simulink library "NeuroMuscularLibrary"  (R2019b)
settings: Solver=ode45  StartTime=0.0  StopTime=10.0  RelTol=1e-3  EnableMultiTasking=on
values from neighbouring files (symbols this model uses):
  a_18_19 = 116    [Prosthesis3R60Params.m]
  a_18_21 = 34    [Prosthesis3R60Params.m]
  a_2_3 = 18    [Prosthesis3R60Params.m]
  angle_offset = 0    [Prosthesis3R60Params.m]
  ankle_height = 0.08    [BodyMechParams.m]
  c = 0.05    [BodyMechParams.m]
  c_jointstop = 0.3 / (pi/180)    (= 17.1887338539)    [BodyMechParams.m]
  c_stance_comp_a0 = 885.0653    [Prosthesis3R60Params.m]
  c_stance_comp_a1 = 2.1443    [Prosthesis3R60Params.m]
  cg14 = 1/2*L14    (= 0.0475)    [Prosthesis3R60Params.m]
  cg25 = (5.45/11.05)*L25    (= 0.0379527149321)    [Prosthesis3R60Params.m]
  cg3 = (3.6/10.4)*L3    (= 0.0306346153846)    [Prosthesis3R60Params.m]
  d_fBall = 0.1    [BodyMechParams.m]
  d_fHeel = 0.05    [BodyMechParams.m]
  deltaLegAngleThr = 8*pi/180    (= 0.13962634016)    [CMGParams.m]
  DeltaThRef = 2e-3    (= 0.002)    [BodyMechParams.m]
  dt_visual = 0.001    [Prosthesis3R60Params.m]
  eref = 0.04    [BodyMechParams.m]
  Fmax = 4000    [MuscleEnergyTest.m]
  FmaxGLU = 1500    [BodyMechParams.m]
  footBallToAnkleDist = 0.16    [BodyMechParams.m]
  footBallToCenterDist = footLength/2    (= 0.1)    [BodyMechParams.m]
  footBallToHeelDist = footLength    (= 0.2)    [BodyMechParams.m]
  footCenterToCGDist = 0.14 - footBallToCenterDist    (= 0.04)    [BodyMechParams.m]
  footInertia = 0.005    [BodyMechParams.m]
  footLength = 0.2    [BodyMechParams.m]
  footMass = 1.25    [BodyMechParams.m]
  FT = 20    [MuscleEnergyTest.m]
  FT_GLU = 47.6    [BodyMechParams.m]
  g = 9.80665    [BodyMechParams.m]
  groundTheta = [atan(diff(groundZ)./diff(groundX)), 0]    [generateGround.m]
  groundZ = groundZ * stepSize/(largestStep+eps)    [generateGround.m]
  hatCenterToCGDist = 0.35 - hatHipToCenterDistLen    (= -0.05)    [BodyMechParams.m]
  hatHipToCenterDistLen = hatLength/2    (= 0.4)    [BodyMechParams.m]
  hatInertia = 3    [BodyMechParams.m]
  hatLeftHipToCenterDistWidth = .15    (= 0.15)    [BodyMechParams.m]
  hatLength = 0.8    [BodyMechParams.m]
  hatMass = 53.5    [BodyMechParams.m]
  hatThickness = 0.2    [BodyMechParams.m]
  hatWidth = 0.4    [BodyMechParams.m]
  J1011 = (4130)*1e-9    (= 4.13e-06)    [Prosthesis3R60Params.m]
  J1415 = (1.18*1e5)*1e-9    (= 0.000118)    [Prosthesis3R60Params.m]
  J18192021 = (6.86*1e4)*1e-9    (= 6.86e-05)    [Prosthesis3R60Params.m]
  J2526 = (3.59*1e4)*1e-9    (= 3.59e-05)    [Prosthesis3R60Params.m]
  J3467 = (25.96*1e4)*1e-9    (= 0.0002596)    [Prosthesis3R60Params.m]
  K = 5    [BodyMechParams.m]
  k_gn = k_gn/2    (= 39226.6)    [BodyMechParams.m]
  k_gt = k_gt/2    (= 39226.6)    [BodyMechParams.m]
  k_pressure = hatMass * g / DeltaThRef    (= 262327.8875)    [BodyMechParams.m]
  k_stance = 130000    [Prosthesis3R60Params.m]
  k_swing = 18750    [Prosthesis3R60Params.m]
  L0_stance = 0.08925    [Prosthesis3R60Params.m]
  L0_swing = 0.0896    [Prosthesis3R60Params.m]
  L10 = 7.9*1e-3    (= 0.0079)    [Prosthesis3R60Params.m]
  L11 = 3.3*1e-3    (= 0.0033)    [Prosthesis3R60Params.m]
  L14 = 95*1e-3    (= 0.095)    [Prosthesis3R60Params.m]
  L15 = 8.2*1e-3    (= 0.0082)    [Prosthesis3R60Params.m]
  L18 = 25.1*1e-3    (= 0.0251)    [Prosthesis3R60Params.m]
  L19 = 17.7*1e-3    (= 0.0177)    [Prosthesis3R60Params.m]
  L20 = 26*1e-3    (= 0.026)    [Prosthesis3R60Params.m]
  L21 = 1.7*1e-3    (= 0.0017)    [Prosthesis3R60Params.m]
  L25 = 76.95*1e-3    (= 0.07695)    [Prosthesis3R60Params.m]
  L26 = 2.8*1e-3    (= 0.0028)    [Prosthesis3R60Params.m]
  L3 = 88.5*1e-3    (= 0.0885)    [Prosthesis3R60Params.m]
  L4 = 1.7*1e-3    (= 0.0017)    [Prosthesis3R60Params.m]
  L6 = 40.25*1e-3    (= 0.04025)    [Prosthesis3R60Params.m]
  L7 = 14.9*1e-3    (= 0.0149)    [Prosthesis3R60Params.m]
  leg_l = [(thighLength - ankle_height/2) (shankLength - ankle_height/2)]    [BodyMechParams.m]
  legAngleSpeedMax = 10    [CMGParams.m]
  lopt = 0.055    [MuscleEnergyTest.m]
  loptBFSH = 0.12    [BodyMechParams.m]
  loptGAS = 0.05    [BodyMechParams.m]
  loptGLU = 0.11    [BodyMechParams.m]
  loptHAB = 0.09    [BodyMechParams.m]
  loptHAD = 0.10    (= 0.1)    [BodyMechParams.m]
  loptHAM = 0.10    (= 0.1)    [BodyMechParams.m]
  loptHFL = 0.11    [BodyMechParams.m]
  loptRF = 0.08    [BodyMechParams.m]
  loptSOL = 0.04    [BodyMechParams.m]
  loptTA = 0.06    [BodyMechParams.m]
  loptVAS = 0.08    [BodyMechParams.m]
  lslack = 0.245    [MuscleEnergyTest.m]
  lslackBFSH = 0.10    (= 0.1)    [BodyMechParams.m]
  lslackGAS = 0.40    (= 0.4)    [BodyMechParams.m]
  lslackGLU = 0.13    [BodyMechParams.m]
  lslackHAB = 0.07    [BodyMechParams.m]
  lslackHAD = 0.18    [BodyMechParams.m]
  lslackHAM = 0.31    [BodyMechParams.m]
  lslackHFL = 0.10    (= 0.1)    [BodyMechParams.m]
  lslackRF = 0.35    [BodyMechParams.m]
  lslackSOL = 0.26    [BodyMechParams.m]
  lslackTA = 0.24    [BodyMechParams.m]
  lslackVAS = 0.23    [BodyMechParams.m]
  m1011 = 49.5*1e-3    (= 0.0495)    [Prosthesis3R60Params.m]
  m1415 = 123.8*1e-3    (= 0.1238)    [Prosthesis3R60Params.m]
  m18192021 = 196.6*1e-3    (= 0.1966)    [Prosthesis3R60Params.m]
  m2526 = 58.3*1e-3    (= 0.0583)    [Prosthesis3R60Params.m]
  m3467 = 253.3*1e-3    (= 0.2533)    [Prosthesis3R60Params.m]
  mu_slide = 0.8    [BodyMechParams.m]
  mu_stick = 0.9    [BodyMechParams.m]
  N = 1.5    [BodyMechParams.m]    (also in cmaes.m = size(x,1); mergeCompareEnergyCosts.m = {S.name})
  phiKneeUpLimit = 5*pi/180    (= 0.0872664625997)    [BodyMechParams.m]
  phimaxGASa = (100-90)*pi/180    (= 0.174532925199)    [BodyMechParams.m]
  phimaxGASk = (180-140)*pi/180    (= 0.698131700798)    [BodyMechParams.m]
  phimaxRFk = (180-165)*pi/180    (= 0.261799387799)    [BodyMechParams.m]
  phimaxSOL = (100-90)*pi/180    (= 0.174532925199)    [BodyMechParams.m]
  phimaxTA = (80-90)*pi/180    (= -0.174532925199)    [BodyMechParams.m]
  phimaxVAS = (180-165)*pi/180    (= 0.261799387799)    [BodyMechParams.m]
  phirefBFSH = (180-160)*pi/180    (= 0.349065850399)    [BodyMechParams.m]
  phirefGASa = (80-90)*pi/180    (= -0.174532925199)    [BodyMechParams.m]
  phirefGASk = (180-165)*pi/180    (= 0.261799387799)    [BodyMechParams.m]
  phirefGLU = (120-180)*pi/180    (= -1.0471975512)    [BodyMechParams.m]
  phirefHAB = 10*pi/180    (= 0.174532925199)    [BodyMechParams.m]
  phirefHAD = 15*pi/180    (= 0.261799387799)    [BodyMechParams.m]
  phirefHAMh = (150-180)*pi/180    (= -0.523598775598)    [BodyMechParams.m]
  phirefHAMk = (180-180)*pi/180    (= 0)    [BodyMechParams.m]
  phirefHFL = (160-180)*pi/180    (= -0.349065850399)    [BodyMechParams.m]
  phirefRFh = (170-180)*pi/180    (= -0.174532925199)    [BodyMechParams.m]
  phirefRFk = (180-125)*pi/180    (= 0.959931088597)    [BodyMechParams.m]
  phirefSOL = (90-90)*pi/180    (= 0)    [BodyMechParams.m]
  ... (+64 more)
undefined symbols (not defined in the file or in its folder): ankleBackDriveGain, ankleCJointstop, ankleDgain, ankleFilterPID, ankleFilterSEA, ankleGearEff, ankleGearRatio, ankleIgain, ankleInitialAngle, ankleInputMass, ankleIntCoulomb, ankleIntDamping, ankleIntStatic, ankleParallelSpringDamping, ankleParallelSpringOffset, ankleParallelSpringStiffness, anklePgain, anklePlantarLimit, ankleSEADamping, ankleSEAStiffness, ankleTendonMass, ankleWMaxJointstop, D12_F, D12_S, D12_T, D12z_T, D13_F, D1G_F, D1G_HAT, D1G_S, D1G_T, D1Gy_F, DeltaS, DeltaSGLU, DeltaSHFL, dryFrictionDamping, dryFrictionStiffness, dryFrictionVelThresh, footMassp, FourBarL1, FourBarL3, GainDphiHATGLUst, GainDphiHATHABst, GainDphiHATHADst, GainDphiHATHFLst, GainFGASst, GainFGLUst, GainFHABst, GainFHAMst, GainFSOLst, GainFSOLTAst, GainFVASst, GainGAS, GainGLU, GainGLUswing, GainHAM, GainHAMHFL ... (+194)
libraries: sm_lib x332, nesl_utility x156, simulink x33, dspswit3 x30, $bdroot x19, simulink_extras x7
(part 7 of 15)

== system NeuroMuscularLibrary/Shanks ==
  CS2_to_knee : sm_lib/Frames and Transforms/Rigid Transform  TranslationMethod=Cartesian  TranslationStandardOffset=0  TranslationLengthUnit=m  TranslationStandardAxis=+Z  TranslationCartesianOffset=[D12_S 0 0]  TranslationROffset=0  TranslationROffsetUnits=m  TranslationZOffset=0  TranslationZOffsetUnits=m  TranslationThetaOffset=0  TranslationThetaOffsetUnits=deg  RotationMethod=None  RotationAngleUnits=deg  RotationStandardAxis=+Z  RotationAngle=0.0  RotationArbitraryAxis=[0 0 1]  FollAlignAxisA=+X  BaseAlignAxisA=+Y  FollAlignAxisB=+Y  BaseAlignAxisB=+Z  RotationSequenceAxes=FollowerAxes  RotationSequence=XYX  RotationSequenceAngles=[0 0 0]  RotationSequenceAnglesUnits=deg  RotationMatrix=[1 0 0; 0 1 0; 0 0 1]
  Cylindrical Solid : sm_lib/Body Elements/Cylindrical Solid  GraphicAmbientColor=[0.15 0.15 0.15 1.0]  BasedOnType=Mass  CenterOfMass=[0 0 0]  CenterOfMassUnits=m  GraphicDiffuseColor=[0.5 0.5 0.5]  CylinderLength=D12_S  CylinderLengthUnits=m  CylinderRadius=.04  CylinderRadiusUnits=m  Density=0  DensityUnits=kg/m^3  DoExposeReferenceFrame=on  GraphicEmissiveColor=[0.0 0.0 0.0 1.0]  ExportEntireGeometry=off  SerializedFrames=<Frames/>  MarkerShape=Sphere  MarkerSize=10  GraphicType=FromGeometry  InertiaType=CalculateFromGeometry  Mass=0  MassUnits=kg  MomentsOfInertia=[1 1 1]  MomentsOfInertiaUnits=kg*m^2  GraphicOpacity=1.0  ProductsOfInertia=[0 0 0]  ProductsOfInertiaUnits=kg*m^2  GraphicShininess=75  GraphicSpecularColor=[0.5 0.5 0.5 1.0]  GraphicVisPropType=SimpleVisualProperties
  Inertia : sm_lib/Body Elements/Inertia  InertiaType=Custom  Mass=m_S  MassUnits=kg  CenterOfMass=[0 0 0]  CenterOfMassUnits=m  MomentsOfInertia=[Inx_S Iny_S In_S]  MomentsOfInertiaUnits=kg*m^2  ProductsOfInertia=[0 0 0]  ProductsOfInertiaUnits=kg*m^2  GraphicType=None  MarkerShape=Inertia  MarkerSize=20  GraphicVisPropType=SimpleVisualProperties  GraphicDiffuseColor=[0.5 0.5 0.5]  GraphicSpecularColor=[0.5 0.5 0.5 1.0]  GraphicAmbientColor=[0.15 0.15 0.15 1.0]  GraphicEmissiveColor=[0.0 0.0 0.0 1.0]  GraphicShininess=75  GraphicOpacity=1.0
  Mux : Mux  Inputs=3
  Mux1 : Mux  Inputs=3
  PS-Simulink Converter{,1..5} (6 alike) : nesl_utility/PS-Simulink Converter  PhysicalDomain=network_engine_domain  SubClassName=ps_output  LeftPortType=input  RightPortType=output  PseudoPeriodic=off  Frequencies=[]  Unit=m  AffineConversion=off
  Reference Frame : sm_lib/Frames and Transforms/Reference Frame
  TO: X-forward Y-up Z-lateral : sm_lib/Frames and Transforms/Rigid Transform  TranslationMethod=StandardAxis  TranslationStandardOffset=D12z_T/2  TranslationLengthUnit=m  TranslationStandardAxis=+Y  TranslationCartesianOffset=[0 0 0]  TranslationROffset=0  TranslationROffsetUnits=m  TranslationZOffset=0  TranslationZOffsetUnits=m  TranslationThetaOffset=0  TranslationThetaOffsetUnits=deg  RotationMethod=AlignedAxes  RotationAngleUnits=deg  RotationStandardAxis=+Z  RotationAngle=0  RotationArbitraryAxis=[0 0 1]  FollAlignAxisA=+Z  BaseAlignAxisA=-Y  FollAlignAxisB=+X  BaseAlignAxisB=+X  RotationSequenceAxes=FollowerAxes  RotationSequence=XYX  RotationSequenceAngles=[0 0 0]  RotationSequenceAnglesUnits=deg  RotationMatrix=[1 0 0; 0 1 0; 0 0 1]
  To CG : sm_lib/Frames and Transforms/Rigid Transform  TranslationMethod=Cartesian  TranslationStandardOffset=0  TranslationLengthUnit=m  TranslationStandardAxis=+Z  TranslationCartesianOffset=[D1G_S 0 0]  TranslationROffset=0  TranslationROffsetUnits=m  TranslationZOffset=0  TranslationZOffsetUnits=m  TranslationThetaOffset=0  TranslationThetaOffsetUnits=deg  RotationMethod=None  RotationAngleUnits=deg  RotationStandardAxis=+Z  RotationAngle=0.0  RotationArbitraryAxis=[0 0 1]  FollAlignAxisA=+X  BaseAlignAxisA=+Y  FollAlignAxisB=+Y  BaseAlignAxisB=+Z  RotationSequenceAxes=FollowerAxes  RotationSequence=XYX  RotationSequenceAngles=[0 0 0]  RotationSequenceAnglesUnits=deg  RotationMatrix=[1 0 0; 0 1 0; 0 0 1]
  To center : sm_lib/Frames and Transforms/Rigid Transform  TranslationMethod=Cartesian  TranslationStandardOffset=0  TranslationLengthUnit=m  TranslationStandardAxis=+Z  TranslationCartesianOffset=[D12_S/2 0 0]  TranslationROffset=0  TranslationROffsetUnits=m  TranslationZOffset=0  TranslationZOffsetUnits=m  TranslationThetaOffset=0  TranslationThetaOffsetUnits=deg  RotationMethod=AlignedAxes  RotationAngleUnits=deg  RotationStandardAxis=+Z  RotationAngle=0.0  RotationArbitraryAxis=[0 0 1]  FollAlignAxisA=+Z  BaseAlignAxisA=+X  FollAlignAxisB=+Y  BaseAlignAxisB=+Y  RotationSequenceAxes=FollowerAxes  RotationSequence=XYX  RotationSequenceAngles=[0 0 0]  RotationSequenceAnglesUnits=deg  RotationMatrix=[1 0 0; 0 1 0; 0 0 1]
  Transform Sensor : sm_lib/Frames and Transforms/Transform Sensor  MeasurementFrame=NonRotatingBase  SenseAngle=off  SenseAxis=off  SenseAngle1=off  SenseAngle2=off  SenseAngle3=off  SenseQ=off  SenseR=off  SenseOmegaX=off  SenseOmegaY=off  SenseOmegaZ=off  SenseOmega1=off  SenseOmega2=off  SenseOmega3=off  SenseQDot=off  SenseRDot=off  SenseAlphaX=off  SenseAlphaY=off  SenseAlphaZ=off  SenseAlpha1=off  SenseAlpha2=off  SenseAlpha3=off  SenseQDDot=off  SenseRDDot=off  SenseX=on  SenseY=on  SenseZ=on  SenseRad=off  SenseAzim=off  SenseDist=off  SenseInc=off  SenseXDot=off  SenseYDot=off  SenseZDot=off  SenseRadDot=off  SenseAzimDot=off  SenseDistDot=off  SenseIncDot=off  SenseXDDot=off  SenseYDDot=off  SenseZDDot=off  SenseRadDDot=off  SenseAzimDDot=off  SenseDistDDot=off  SenseIncDDot=off
  Transform Sensor1 : sm_lib/Frames and Transforms/Transform Sensor  MeasurementFrame=NonRotatingBase  SenseAngle=off  SenseAxis=off  SenseAngle1=off  SenseAngle2=off  SenseAngle3=off  SenseQ=off  SenseR=off  SenseOmegaX=off  SenseOmegaY=off  SenseOmegaZ=off  SenseOmega1=off  SenseOmega2=off  SenseOmega3=off  SenseQDot=off  SenseRDot=off  SenseAlphaX=off  SenseAlphaY=off  SenseAlphaZ=off  SenseAlpha1=off  SenseAlpha2=off  SenseAlpha3=off  SenseQDDot=off  SenseRDDot=off  SenseX=on  SenseY=on  SenseZ=on  SenseRad=off  SenseAzim=off  SenseDist=off  SenseInc=off  SenseXDot=off  SenseYDot=off  SenseZDot=off  SenseRadDot=off  SenseAzimDot=off  SenseDistDot=off  SenseIncDot=off  SenseXDDot=off  SenseYDDot=off  SenseZDDot=off  SenseRadDDot=off  SenseAzimDDot=off  SenseDistDDot=off  SenseIncDDot=off
  World Frame1 : sm_lib/Frames and Transforms/World Frame
  Ankle : PMIOPort  Side=Right
  Knee : PMIOPort  Port=2  Side=Left
  Ankle pos : Outport
  CG pos : Outport  Port=2
  wires:
  Mux/1 -> Ankle pos/1
  PS-Simulink Converter1/1 -> Mux/3
  PS-Simulink Converter2/1 -> Mux/2
  PS-Simulink Converter/1 -> Mux/1
  PS-Simulink Converter3/1 -> Mux1/1
  PS-Simulink Converter4/1 -> Mux1/2
  PS-Simulink Converter5/1 -> Mux1/3
  Mux1/1 -> CG pos/1
  connections:
  TO: X-forward Y-up Z-lateral/RConn1 -- Reference Frame/RConn1 -- Transform Sensor1/LConn1 -- Transform Sensor/LConn1
  Transform Sensor/RConn4 -- PS-Simulink Converter1/LConn1
  Transform Sensor/RConn3 -- PS-Simulink Converter2/LConn1
  PS-Simulink Converter/LConn1 -- Transform Sensor/RConn2
  To CG/LConn1 -- To center/LConn1 -- Transform Sensor/RConn1 -- Ankle/RConn1 -- CS2_to_knee/LConn1
  To CG/RConn1 -- Inertia/RConn1 -- Transform Sensor1/RConn1
  Knee/RConn1 -- CS2_to_knee/RConn1
  To center/RConn1 -- Cylindrical Solid/RConn1
  TO: X-forward Y-up Z-lateral/LConn1 -- World Frame1/RConn1
  Transform Sensor1/RConn4 -- PS-Simulink Converter5/LConn1
  Transform Sensor1/RConn3 -- PS-Simulink Converter4/LConn1
  Transform Sensor1/RConn2 -- PS-Simulink Converter3/LConn1

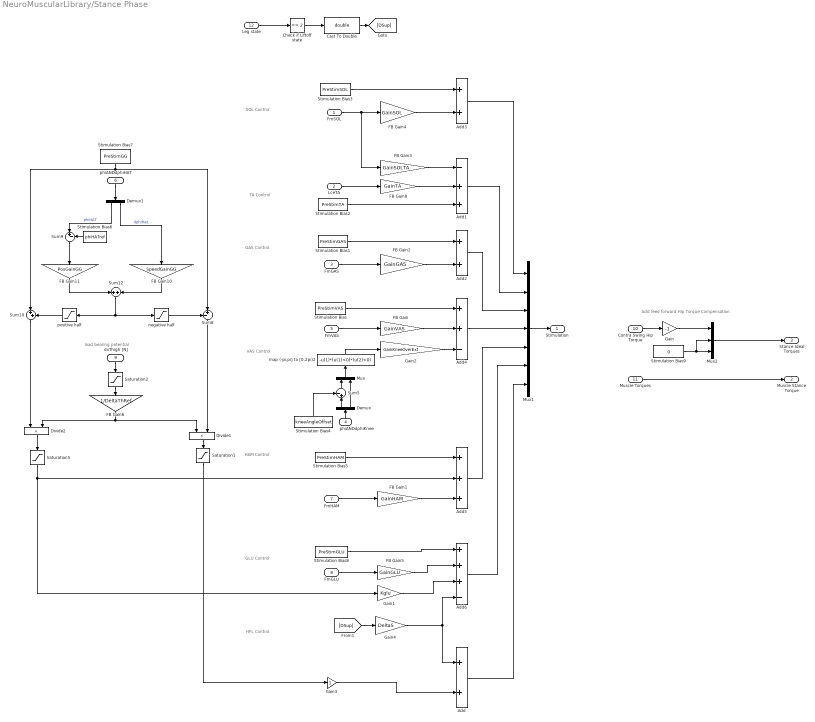
== system NeuroMuscularLibrary/Stance Phase ==
  note: SOL Control
  note: TA Control
  note: GAS Control
  note: HAM Control
  note: VAS Control
  note: GLU Control
  note: HFL Control
  note: load bearing potential
  note: Add feed forward Hip Torque Compensation
  FmSOL : Inport
  LceTA : Inport  Port=2
  FmGAS : Inport  Port=3
  phiANDdphiKnee : Inport  Port=4
  FmVAS : Inport  Port=5
  phiANDdphiHAT : Inport  Port=6
  FmHAM : Inport  Port=7
  FmGLU : Inport  Port=8
  dxThigh [N] : Inport  Port=9
  Contra Swing Hip Torque : Inport  Port=10
  Muscle Torques : Inport  Port=11
  Leg state : Inport  Port=12
  Add : Sum
  Add1 : Sum  Inputs=-++
  Add2 : Sum
  Add3 : Sum
  Add4 : Sum  Inputs=++-
  Add5 : Sum  Inputs=+++
  Add6 : Sum  Inputs=+++-
  Cast To Double : DataTypeConversion  OutDataTypeStr=double
  Check if Liftoff state : simulink/Logic and Bit Operations/Compare To Constant  relop===  const=2  OutDataTypeStr=boolean
  Demux : Demux  Outputs=2
  Demux1 : Demux  Outputs=2
  Divide1 : Product
  Divide2 : Product
  FB Gain : Gain  Gain=GainVAS  SaturateOnIntegerOverflow=on  OutDataTypeStr=Inherit: Same as input  ParamDataTypeStr=Inherit: Same as input
  FB Gain1 : Gain  Gain=GainHAM  SaturateOnIntegerOverflow=on  OutDataTypeStr=Inherit: Same as input  ParamDataTypeStr=Inherit: Same as input
  FB Gain10 : Gain  Gain=SpeedGainGG  SaturateOnIntegerOverflow=on  OutDataTypeStr=Inherit: Same as input  ParamDataTypeStr=Inherit: Same as input
  FB Gain11 : Gain  Gain=PosGainGG  SaturateOnIntegerOverflow=on  OutDataTypeStr=Inherit: Same as input  ParamDataTypeStr=Inherit: Same as input
  FB Gain2 : Gain  Gain=GainGAS  SaturateOnIntegerOverflow=on  OutDataTypeStr=Inherit: Same as input  ParamDataTypeStr=Inherit: Same as input
  FB Gain3 : Gain  Gain=GainSOLTA  SaturateOnIntegerOverflow=on  OutDataTypeStr=Inherit: Same as input  ParamDataTypeStr=Inherit: Same as input
  FB Gain4 : Gain  Gain=GainSOL  SaturateOnIntegerOverflow=on  OutDataTypeStr=Inherit: Same as input  ParamDataTypeStr=Inherit: Same as input
  FB Gain5 : Gain  Gain=GainGLU  SaturateOnIntegerOverflow=on  OutDataTypeStr=Inherit: Same as input  ParamDataTypeStr=Inherit: Same as input
  FB Gain6 : Gain  Gain=1/DeltaThRef  SaturateOnIntegerOverflow=on  OutDataTypeStr=Inherit: Same as input  ParamDataTypeStr=Inherit: Same as input
  FB Gain8 : Gain  Gain=GainTA  SaturateOnIntegerOverflow=on  OutDataTypeStr=Inherit: Same as input  ParamDataTypeStr=Inherit: Same as input
  Gain : Gain  Gain=-1
  Gain1 : Gain  Gain=Kglu
  Gain2 : Gain  Gain=GainKneeOverExt
  Gain3 : Gain
  Gain4 : Gain  Gain=DeltaS
  Mux : Mux  Inputs=2
  Mux1 : Mux  Inputs=7
  Mux2 : Mux  Inputs=3
  Saturation1 : Saturate  UpperLimit=1  LowerLimit=0  ZeroCross=off
  Saturation2 : Saturate  UpperLimit=inf  LowerLimit=0  ZeroCross=off
  Saturation5 : Saturate  UpperLimit=1  LowerLimit=0  ZeroCross=off
  Stimulation Bias : Constant  Value=PreStimVAS
  Stimulation Bias1 : Constant  Value=PreStimGAS
  Stimulation Bias2 : Constant  Value=PreStimTA
  Stimulation Bias3 : Constant  Value=PreStimSOL
  Stimulation Bias4 : Constant  Value=kneeAngleOffset
  Stimulation Bias5 : Constant  Value=PreStimHAM
  Stimulation Bias6 : Constant  Value=phiHATref
  Stimulation Bias7 : Constant  Value=PreStimGG
  Stimulation Bias8 : Constant  Value=PreStimGLU
  Stimulation Bias9 : Constant  Value=0
  Sum10 : Sum  Inputs=|++  SaturateOnIntegerOverflow=on  InputSameDT=on  OutDataTypeStr=Inherit: Same as first input
  Sum12 : Sum  SaturateOnIntegerOverflow=on  InputSameDT=on  OutDataTypeStr=Inherit: Same as first input
  Sum5 : Sum  Inputs=-+|  SaturateOnIntegerOverflow=on  InputSameDT=on  OutDataTypeStr=Inherit: Same as first input
  Sum8 : Sum  Inputs=-+|  SaturateOnIntegerOverflow=on  InputSameDT=on  OutDataTypeStr=Inherit: Same as first input
  Sum9 : Sum  Inputs=|+-  SaturateOnIntegerOverflow=on  InputSameDT=on  OutDataTypeStr=Inherit: Same as first input
  map (-pi,pi] to [0,2pi)2 : Fcn  Expr=-u(1)*(u(1)<0)*(u(2)<0)
  negative half : Saturate  UpperLimit=0  LowerLimit=-inf  ZeroCross=off
  positive half : Saturate  UpperLimit=inf  LowerLimit=0  ZeroCross=off
  Stimulation : Outport
  Muscle Stance Torque : Outport  Port=2
  Stance Ideal Torques : Outport  Port=3
  wires:
  Muscle Torques/1 -> Muscle Stance Torque/1
  Mux2/1 -> Stance Ideal Torques/1
  Stimulation Bias9/1 -> Mux2/2, Mux2/3
  Add3/1 -> Mux1/1
  FB Gain4/1 -> Add3/2
  FmSOL/1 -> FB Gain4/1, FB Gain3/1
  FB Gain3/1 -> Add1/1
  Add1/1 -> Mux1/2
  FB Gain8/1 -> Add1/2
  LceTA/1 -> FB Gain8/1
  FmGAS/1 -> FB Gain2/1
  FB Gain2/1 -> Add2/2
  FB Gain/1 -> Add4/2
  FmVAS/1 -> FB Gain/1
  Mux/1 -> map (-pi,pi] to [0,2pi)2/1
  Sum5/1 -> Mux/1
  phiANDdphiKnee/1 -> Demux/1
  Demux/1 -> Sum5/2
  Demux/2 -> Mux/2
  Stimulation Bias4/1 -> Sum5/1
  Stimulation Bias6/1 -> Sum9/2
  Stimulation Bias7/1 -> Sum10/1, Sum8/2
  FB Gain11/1 -> Sum12/1
  FB Gain10/1 -> Sum12/2
  phiANDdphiHAT/1 -> Demux1/1
  Demux1/1 -> Sum9/1  "phiHAT"
  Demux1/2 -> FB Gain10/1  "dphiHat"
  positive half/1 -> Sum10/2
  Sum12/1 -> positive half/1, negative half/1
  negative half/1 -> Sum8/1
  Gain2/1 -> Add4/3
  Add/1 -> Mux1/7
  Saturation2/1 -> FB Gain6/1
  dxThigh [N]/1 -> Saturation2/1
  Saturation1/1 -> Gain3/1
  Divide1/1 -> Saturation1/1
  Divide2/1 -> Saturation5/1
  Saturation5/1 -> Gain1/1, Add5/2
  FB Gain6/1 -> Divide2/2, Divide1/1
  Sum9/1 -> FB Gain11/1
  Sum10/1 -> Divide2/1
  Sum8/1 -> Divide1/2
  map (-pi,pi] to [0,2pi)2/1 -> Gain2/1
  FmHAM/1 -> FB Gain1/1
  FmGLU/1 -> FB Gain5/1
  Stimulation Bias3/1 -> Add3/1
  Stimulation Bias2/1 -> Add1/3
  Add2/1 -> Mux1/3
  Stimulation Bias1/1 -> Add2/1
  Stimulation Bias/1 -> Add4/1
  Stimulation Bias5/1 -> Add5/1
  FB Gain1/1 -> Add5/3
  Add5/1 -> Mux1/5
  Add6/1 -> Mux1/6
  Stimulation Bias8/1 -> Add6/1
  FB Gain5/1 -> Add6/2
  Gain1/1 -> Add6/3
  Mux1/1 -> Stimulation/1
  Add4/1 -> Mux1/4
  Contra Swing Hip Torque/1 -> Gain/1
  Gain/1 -> Mux2/1
  Cast To Double/1 -> [DSup]
  Check if Liftoff state/1 -> Cast To Double/1
  Leg state/1 -> Check if Liftoff state/1
  Gain3/1 -> Add/2
  [DSup] -> Gain4/1
  Gain4/1 -> Add6/4, Add/1

== system NeuroMuscularLibrary/Stance Phase (coronal) ==
  note: Stance Phase Control
  note: M3: balance trunk
  note: M4: compensate swing leg
  phiHATref : Inport
  phi dphi [rad rad/s] : Inport  Port=2
  CSwingStim : Inport  Port=3
  FmHAB : Inport  Port=4
  Enable : EnablePort  StatesWhenEnabling=reset  ZeroCross=off
  " 1" : Gain  Gain=GainPhiHATHABst
  " 2" : Gain  Gain=GainDphiHATHABst
  " 3" : Gain  Gain=GainFHABst
  " 4" : Gain  Gain=GainPhiHATHADst
  " 5" : Gain  Gain=GainDphiHATHADst
  " 6" : Gain  Gain=GainSHABcHABst
  " 7" : Gain  Gain=GainSHADcHADst
  Constant12 : Constant  Value=PreStimHADst
  Constant15 : Constant  Value=PreStimHABst
  Demux7 : Demux  Outputs=2
  Demux8 : Demux  Outputs=2
  Gain2 : Gain  Gain=-1
  Gain3 : Gain  Gain=-1
  Mux : Mux  Inputs=2
  Mux1 : Mux  Inputs=2
  Mux2 : Mux  Inputs=2
  Sum4 : Sum  Inputs=-+|  SaturateOnIntegerOverflow=on  InputSameDT=on  OutDataTypeStr=Inherit: Same as first input
  Sum5 : Sum  SaturateOnIntegerOverflow=on  InputSameDT=on  OutDataTypeStr=Inherit: Same as first input
  Sum6 : Sum  SaturateOnIntegerOverflow=on  InputSameDT=on  OutDataTypeStr=Inherit: Same as first input
  positive half1 : Saturate  UpperLimit=inf  LowerLimit=0  ZeroCross=off
  positive half2 : Saturate  UpperLimit=inf  LowerLimit=0  ZeroCross=off
  S_0_St : Outport  OutputWhenDisabled=reset  InitialOutput=0
  S_M1 [HAB] : Outport  Port=2  OutputWhenDisabled=reset  InitialOutput=0
  S_M3 [HAB HAD] : Outport  Port=3  OutputWhenDisabled=reset  InitialOutput=0
  S_M4 [HAB HAD] : Outport  Port=4  OutputWhenDisabled=reset  InitialOutput=0
  wires:
  phi dphi [rad rad/s]/1 -> Demux7/1
  Demux7/1 -> Sum4/2  "theta"
  Demux7/2 -> " 5"/1, Gain3/1  "dtheta"
  phiHATref/1 -> Sum4/1
  Sum4/1 -> " 4"/1, Gain2/1
  Gain2/1 -> " 1"/1
  Gain3/1 -> " 2"/1
  " 1"/1 -> Sum5/1
  " 2"/1 -> Sum5/2
  " 4"/1 -> Sum6/1
  " 5"/1 -> Sum6/2
  Sum5/1 -> positive half1/1  "HAB"
  Sum6/1 -> positive half2/1  "HAD"
  Mux1/1 -> S_M3 [HAB HAD]/1
  Mux/1 -> S_0_St/1
  CSwingStim/1 -> Demux8/1
  Mux2/1 -> S_M4 [HAB HAD]/1
  Demux8/1 -> " 6"/1  "Stim_CHAB"
  Demux8/2 -> " 7"/1  "Stim_CHAD"
  " 6"/1 -> Mux2/1  "HAB"
  " 7"/1 -> Mux2/2  "HAD"
  positive half1/1 -> Mux1/1
  positive half2/1 -> Mux1/2
  " 3"/1 -> S_M1 [HAB]/1  "HAB"
  FmHAB/1 -> " 3"/1
  Constant12/1 -> Mux/2
  Constant15/1 -> Mux/1

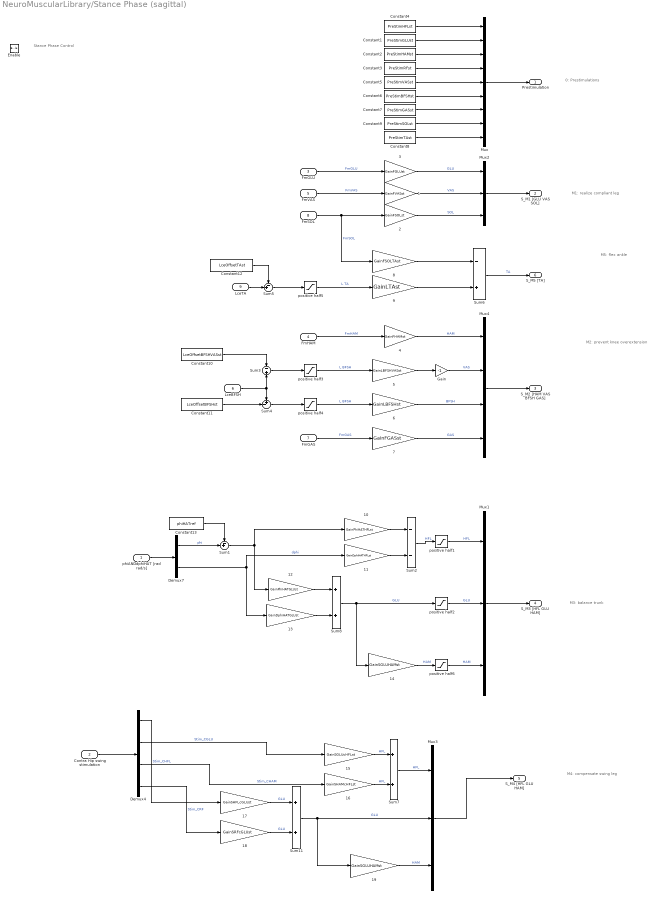
== system NeuroMuscularLibrary/Stance Phase (sagittal) ==
  note: M4: compensate swing leg
  note: M3: balance trunk
  note: M5: flex ankle
  note: M2: prevent knee overextension
  note: M1: realize compliant leg
  note: 0: Prestimulations
  note: Stance Phase Control
  phiANDdphiHAT [rad rad/s] : Inport
  Contra Hip swing stimulation : Inport  Port=2
  FmGLU : Inport  Port=3
  FmHAM : Inport  Port=4
  FmVAS : Inport  Port=5
  LceBFSH : Inport  Port=6
  FmGAS : Inport  Port=7
  FmSOL : Inport  Port=8
  LceTA : Inport  Port=9
  Enable : EnablePort  StatesWhenEnabling=reset  ZeroCross=off
  " 1" : Gain  Gain=GainFVASst
  " 10" : Gain  Gain=GainPhiHATHFLst
  " 11" : Gain  Gain=GainDphiHATHFLst
  " 12" : Gain  Gain=GainPhiHATGLUst
  " 13" : Gain  Gain=GainDphiHATGLUst
  " 14" : Gain  Gain=GainSGLUHAMst
  " 15" : Gain  Gain=GainSGLUcHFLst
  " 16" : Gain  Gain=GainSHAMcHFLst
  " 17" : Gain  Gain=GainSHFLcGLUst
  " 18" : Gain  Gain=GainSRFcGLUst
  " 19" : Gain  Gain=GainSGLUHAMst
  " 2" : Gain  Gain=GainFSOLst
  " 3" : Gain  Gain=GainFGLUst
  " 4" : Gain  Gain=GainFHAMst
  " 5" : Gain  Gain=GainLBFSHVASst
  " 6" : Gain  Gain=GainLBFSHst
  " 7" : Gain  Gain=GainFGASst
  " 8" : Gain  Gain=GainFSOLTAst
  " 9" : Gain  Gain=GainLTAst
  Constant1 : Constant  Value=PreStimGLUst
  Constant10 : Constant  Value=LceOffsetBFSHVASst
  Constant11 : Constant  Value=LceOffsetBFSHst
  Constant12 : Constant  Value=LceOffsetTAst
  Constant13 : Constant  Value=phiHATref
  Constant2 : Constant  Value=PreStimHAMst
  Constant3 : Constant  Value=PreStimRFst
  Constant4 : Constant  Value=PreStimHFLst
  Constant5 : Constant  Value=PreStimVASst
  Constant6 : Constant  Value=PreStimBFSHst
  Constant7 : Constant  Value=PreStimGASst
  Constant8 : Constant  Value=PreStimTAst
  Constant9 : Constant  Value=PreStimSOLst
  Demux4 : Demux
  Demux7 : Demux  Outputs=2
  Gain : Gain  Gain=-1
  Mux : Mux  Inputs=9
  Mux1 : Mux  Inputs=3
  Mux2 : Mux  Inputs=3
  Mux3 : Mux  Inputs=3
  Mux4 : Mux
  Sum1 : Sum  Inputs=-+|  SaturateOnIntegerOverflow=on  InputSameDT=on  OutDataTypeStr=Inherit: Same as first input
  Sum11 : Sum  SaturateOnIntegerOverflow=on  InputSameDT=on  OutDataTypeStr=Inherit: Same as first input
  Sum2 : Sum  Inputs=--  SaturateOnIntegerOverflow=on  InputSameDT=on  OutDataTypeStr=Inherit: Same as first input
  Sum3 : Sum  Inputs=-|+  SaturateOnIntegerOverflow=on  InputSameDT=on  OutDataTypeStr=Inherit: Same as first input
  Sum4 : Sum  Inputs=+-|  SaturateOnIntegerOverflow=on  InputSameDT=on  OutDataTypeStr=Inherit: Same as first input
  Sum5 : Sum  Inputs=-+|  SaturateOnIntegerOverflow=on  InputSameDT=on  OutDataTypeStr=Inherit: Same as first input
  Sum6 : Sum  Inputs=-+  SaturateOnIntegerOverflow=on  InputSameDT=on  OutDataTypeStr=Inherit: Same as first input
  Sum7 : Sum  SaturateOnIntegerOverflow=on  InputSameDT=on  OutDataTypeStr=Inherit: Same as first input
  Sum8 : Sum  SaturateOnIntegerOverflow=on  InputSameDT=on  OutDataTypeStr=Inherit: Same as first input
  positive half{1..6} (6 alike) : Saturate  UpperLimit=inf  LowerLimit=0  ZeroCross=off
  Prestimulation : Outport  OutputWhenDisabled=reset  InitialOutput=0
  S_M1 [GLU VAS SOL] : Outport  Port=2  OutputWhenDisabled=reset  InitialOutput=0
  S_M2 [HAM VAS BFSH GAS] : Outport  Port=3  OutputWhenDisabled=reset  InitialOutput=0
  S_M3 [HFL GLU HAM] : Outport  Port=4  OutputWhenDisabled=reset  InitialOutput=0
  S_M4 [HFL GLU HAM] : Outport  Port=5  OutputWhenDisabled=reset  InitialOutput=0
  S_M5 [TA] : Outport  Port=6  OutputWhenDisabled=reset  InitialOutput=0
  wires:
  Sum11/1 -> " 19"/1, Mux3/2  "GLU"
  Sum7/1 -> Mux3/1  "HFL"
  Demux4/4 -> " 18"/1  "Stim_CRF"
  Demux4/3 -> " 16"/1  "Stim_CHAM"
  Mux3/1 -> S_M4 [HFL GLU HAM]/1
  Demux4/2 -> " 15"/1  "Stim_CGLU"
  Demux4/1 -> " 17"/1  "Stim_CHFL"
  Contra Hip swing stimulation/1 -> Demux4/1
  positive half6/1 -> Mux1/3  "HAM"
  positive half2/1 -> Mux1/2  "GLU"
  positive half1/1 -> Mux1/1  "HFL"
  Constant13/1 -> Sum1/1
  " 14"/1 -> positive half6/1  "HAM"
  Mux1/1 -> S_M3 [HFL GLU HAM]/1
  Sum8/1 -> " 14"/1, positive half2/1  "GLU"
  Sum2/1 -> positive half1/1  "HFL"
  " 13"/1 -> Sum8/2
  " 12"/1 -> Sum8/1
  " 11"/1 -> Sum2/2
  " 10"/1 -> Sum2/1
  Sum1/1 -> " 10"/1, " 12"/1
  Demux7/2 -> " 11"/1, " 13"/1  "dphi"
  Demux7/1 -> Sum1/2  "phi"
  phiANDdphiHAT [rad rad/s]/1 -> Demux7/1
  Mux4/1 -> S_M2 [HAM VAS BFSH GAS]/1
  LceTA/1 -> Sum5/2
  Sum6/1 -> S_M5 [TA]/1  "TA"
  " 8"/1 -> Sum6/1
  positive half5/1 -> " 9"/1  "L TA"
  Sum5/1 -> positive half5/1
  LceBFSH/1 -> Sum3/2, Sum4/1
  Sum4/1 -> positive half4/1
  Gain/1 -> Mux4/2  "VAS"
  FmHAM/1 -> " 4"/1  "FmHAM"
  FmGAS/1 -> " 7"/1  "FmGAS"
  positive half4/1 -> " 6"/1  "L BFSH"
  positive half3/1 -> " 5"/1  "L BFSH"
  Sum3/1 -> positive half3/1
  Mux2/1 -> S_M1 [GLU VAS SOL]/1
  FmGLU/1 -> " 3"/1  "FmGLU"
  FmVAS/1 -> " 1"/1  "FmVAS"
  FmSOL/1 -> " 8"/1, " 2"/1  "FmSOL"
  Constant4/1 -> Mux/1
  Constant1/1 -> Mux/2
  Constant2/1 -> Mux/3
  Constant3/1 -> Mux/4
  Constant5/1 -> Mux/5
  Constant6/1 -> Mux/6
  Constant7/1 -> Mux/7
  Constant8/1 -> Mux/9
  Constant9/1 -> Mux/8
  Mux/1 -> Prestimulation/1
  " 3"/1 -> Mux2/1  "GLU"
  " 1"/1 -> Mux2/2  "VAS"
  " 2"/1 -> Mux2/3  "SOL"
  " 4"/1 -> Mux4/1  "HAM"
  Constant10/1 -> Sum3/1
  " 5"/1 -> Gain/1
  Constant11/1 -> Sum4/2
  " 6"/1 -> Mux4/3  "BFSH"
  " 7"/1 -> Mux4/4  "GAS"
  Constant12/1 -> Sum5/1
  " 9"/1 -> Sum6/2
  " 19"/1 -> Mux3/3  "HAM"
  " 15"/1 -> Sum7/1  "HFL"
  " 16"/1 -> Sum7/2  "HFL"
  " 17"/1 -> Sum11/1  "GLU"
  " 18"/1 -> Sum11/2  "GLU"

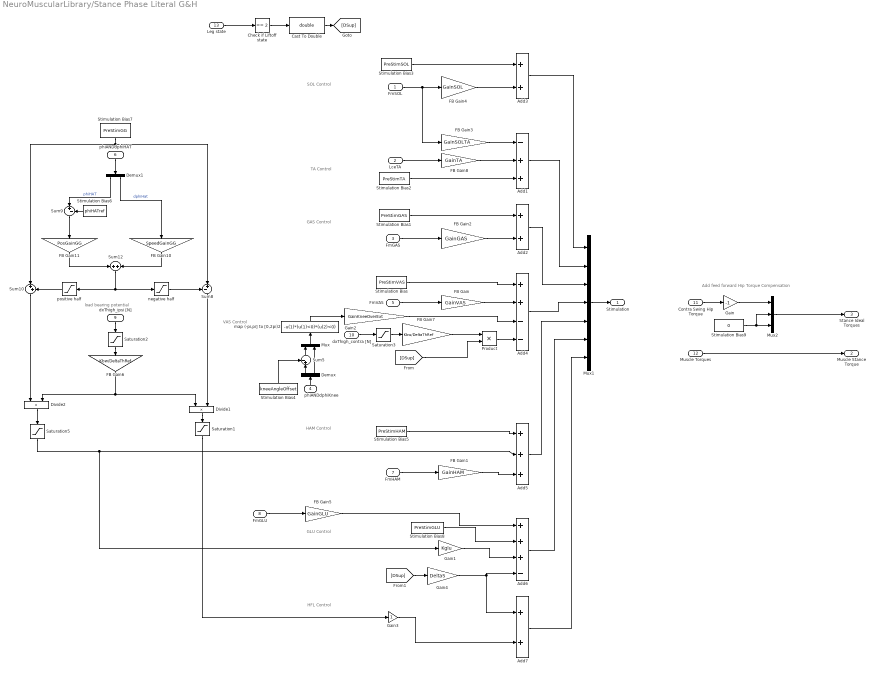
== system NeuroMuscularLibrary/Stance Phase Literal G&H ==
  note: Add feed forward Hip Torque Compensation
  note: load bearing potential
  note: HFL Control
  note: GLU Control
  note: VAS Control
  note: HAM Control
  note: GAS Control
  note: TA Control
  note: SOL Control
  FmSOL : Inport
  LceTA : Inport  Port=2
  FmGAS : Inport  Port=3
  phiANDdphiKnee : Inport  Port=4
  FmVAS : Inport  Port=5
  phiANDdphiHAT : Inport  Port=6
  FmHAM : Inport  Port=7
  FmGLU : Inport  Port=8
  dxThigh_ipsi [N] : Inport  Port=9
  dxThigh_contra [N] : Inport  Port=10
  Contra Swing Hip Torque : Inport  Port=11
  Muscle Torques : Inport  Port=12
  Leg state : Inport  Port=13
  Add1 : Sum  Inputs=-++
  Add2 : Sum
  Add3 : Sum
  Add4 : Sum  Inputs=++--
  Add5 : Sum  Inputs=+++
  Add6 : Sum  Inputs=+++-
  Add7 : Sum
  Cast To Double : DataTypeConversion  OutDataTypeStr=double
  Check if Liftoff state : simulink/Logic and Bit Operations/Compare To Constant  relop===  const=2  OutDataTypeStr=boolean
  Demux : Demux  Outputs=2
  Demux1 : Demux  Outputs=2
  Divide1 : Product
  Divide2 : Product
  FB Gain : Gain  Gain=GainVAS  SaturateOnIntegerOverflow=on  OutDataTypeStr=Inherit: Same as input  ParamDataTypeStr=Inherit: Same as input
  FB Gain1 : Gain  Gain=GainHAM  SaturateOnIntegerOverflow=on  OutDataTypeStr=Inherit: Same as input  ParamDataTypeStr=Inherit: Same as input
  FB Gain10 : Gain  Gain=SpeedGainGG  SaturateOnIntegerOverflow=on  OutDataTypeStr=Inherit: Same as input  ParamDataTypeStr=Inherit: Same as input
  FB Gain11 : Gain  Gain=PosGainGG  SaturateOnIntegerOverflow=on  OutDataTypeStr=Inherit: Same as input  ParamDataTypeStr=Inherit: Same as input
  FB Gain2 : Gain  Gain=GainGAS  SaturateOnIntegerOverflow=on  OutDataTypeStr=Inherit: Same as input  ParamDataTypeStr=Inherit: Same as input
  FB Gain3 : Gain  Gain=GainSOLTA  SaturateOnIntegerOverflow=on  OutDataTypeStr=Inherit: Same as input  ParamDataTypeStr=Inherit: Same as input
  FB Gain4 : Gain  Gain=GainSOL  SaturateOnIntegerOverflow=on  OutDataTypeStr=Inherit: Same as input  ParamDataTypeStr=Inherit: Same as input
  FB Gain5 : Gain  Gain=GainGLU  SaturateOnIntegerOverflow=on  OutDataTypeStr=Inherit: Same as input  ParamDataTypeStr=Inherit: Same as input
  FB Gain6 : Gain  Gain=Kbw/DeltaThRef  SaturateOnIntegerOverflow=on  OutDataTypeStr=Inherit: Same as input  ParamDataTypeStr=Inherit: Same as input
  FB Gain7 : Gain  Gain=Kbw/DeltaThRef  SaturateOnIntegerOverflow=on  OutDataTypeStr=Inherit: Same as input  ParamDataTypeStr=Inherit: Same as input
  FB Gain8 : Gain  Gain=GainTA  SaturateOnIntegerOverflow=on  OutDataTypeStr=Inherit: Same as input  ParamDataTypeStr=Inherit: Same as input
  Gain : Gain  Gain=-1
  Gain1 : Gain  Gain=Kglu
  Gain2 : Gain  Gain=GainKneeOverExt
  Gain3 : Gain
  Gain4 : Gain  Gain=DeltaS
  Mux : Mux  Inputs=2
  Mux1 : Mux  Inputs=7
  Mux2 : Mux  Inputs=3
  Product : Product
  Saturation1 : Saturate  UpperLimit=1  LowerLimit=0  ZeroCross=off
  Saturation2 : Saturate  UpperLimit=inf  LowerLimit=0  ZeroCross=off
  Saturation3 : Saturate  UpperLimit=inf  LowerLimit=0  ZeroCross=off
  Saturation5 : Saturate  UpperLimit=1  LowerLimit=0  ZeroCross=off
  Stimulation Bias : Constant  Value=PreStimVAS
  Stimulation Bias1 : Constant  Value=PreStimGAS
  Stimulation Bias2 : Constant  Value=PreStimTA
  Stimulation Bias3 : Constant  Value=PreStimSOL
  Stimulation Bias4 : Constant  Value=kneeAngleOffset
  Stimulation Bias5 : Constant  Value=PreStimHAM
  Stimulation Bias6 : Constant  Value=phiHATref
  Stimulation Bias7 : Constant  Value=PreStimGG
  Stimulation Bias8 : Constant  Value=PreStimGLU
  Stimulation Bias9 : Constant  Value=0
  Sum10 : Sum  Inputs=|++  SaturateOnIntegerOverflow=on  InputSameDT=on  OutDataTypeStr=Inherit: Same as first input
  Sum12 : Sum  SaturateOnIntegerOverflow=on  InputSameDT=on  OutDataTypeStr=Inherit: Same as first input
  Sum5 : Sum  Inputs=-+|  SaturateOnIntegerOverflow=on  InputSameDT=on  OutDataTypeStr=Inherit: Same as first input
  Sum8 : Sum  Inputs=-+|  SaturateOnIntegerOverflow=on  InputSameDT=on  OutDataTypeStr=Inherit: Same as first input
  Sum9 : Sum  Inputs=|+-  SaturateOnIntegerOverflow=on  InputSameDT=on  OutDataTypeStr=Inherit: Same as first input
  map (-pi,pi] to [0,2pi)2 : Fcn  Expr=-u(1)*(u(1)<0)*(u(2)<0)
  negative half : Saturate  UpperLimit=0  LowerLimit=-inf  ZeroCross=off
  positive half : Saturate  UpperLimit=inf  LowerLimit=0  ZeroCross=off
  Stimulation : Outport
  Muscle Stance Torque : Outport  Port=2
  Stance Ideal Torques : Outport  Port=3
  wires:
  Gain/1 -> Mux2/1
  Contra Swing Hip Torque/1 -> Gain/1
  Add4/1 -> Mux1/4
  Mux1/1 -> Stimulation/1
  FB Gain5/1 -> Add6/1
  Stimulation Bias8/1 -> Add6/2
  Add6/1 -> Mux1/6
  Saturation5/1 -> Add5/2, Gain1/1
  FB Gain1/1 -> Add5/3
  Stimulation Bias5/1 -> Add5/1
  Stimulation Bias/1 -> Add4/1
  Stimulation Bias1/1 -> Add2/1
  Add2/1 -> Mux1/3
  Stimulation Bias2/1 -> Add1/3
  Stimulation Bias3/1 -> Add3/1
  FmGLU/1 -> FB Gain5/1
  FmHAM/1 -> FB Gain1/1
  map (-pi,pi] to [0,2pi)2/1 -> Gain2/1
  Sum8/1 -> Divide1/2
  Sum10/1 -> Divide2/1
  Sum9/1 -> FB Gain11/1
  FB Gain6/1 -> Divide1/1, Divide2/2
  Divide2/1 -> Saturation5/1
  Divide1/1 -> Saturation1/1
  Saturation1/1 -> Gain3/1
  dxThigh_ipsi [N]/1 -> Saturation2/1
  Saturation2/1 -> FB Gain6/1
  Add7/1 -> Mux1/7
  Gain2/1 -> Add4/3
  negative half/1 -> Sum8/1
  Sum12/1 -> negative half/1, positive half/1
  positive half/1 -> Sum10/2
  Demux1/2 -> FB Gain10/1  "dphiHat"
  Demux1/1 -> Sum9/1  "phiHAT"
  phiANDdphiHAT/1 -> Demux1/1
  FB Gain10/1 -> Sum12/2
  FB Gain11/1 -> Sum12/1
  Stimulation Bias7/1 -> Sum8/2, Sum10/1
  Stimulation Bias6/1 -> Sum9/2
  Stimulation Bias4/1 -> Sum5/1
  Demux/2 -> Mux/2
  Demux/1 -> Sum5/2
  phiANDdphiKnee/1 -> Demux/1
  Sum5/1 -> Mux/1
  Mux/1 -> map (-pi,pi] to [0,2pi)2/1
  FmVAS/1 -> FB Gain/1
  FB Gain/1 -> Add4/2
  FB Gain2/1 -> Add2/2
  FmGAS/1 -> FB Gain2/1
  LceTA/1 -> FB Gain8/1
  FB Gain8/1 -> Add1/2
  Add1/1 -> Mux1/2
  FB Gain3/1 -> Add1/1
  FmSOL/1 -> FB Gain3/1, FB Gain4/1
  FB Gain4/1 -> Add3/2
  Add3/1 -> Mux1/1
  Stimulation Bias9/1 -> Mux2/3, Mux2/2
  Mux2/1 -> Stance Ideal Torques/1
  Muscle Torques/1 -> Muscle Stance Torque/1
  dxThigh_contra [N]/1 -> Saturation3/1
  Saturation3/1 -> FB Gain7/1
  FB Gain7/1 -> Product/1
  Check if Liftoff state/1 -> Cast To Double/1
  Leg state/1 -> Check if Liftoff state/1
  [DSup] -> Product/2
  Product/1 -> Add4/4
  Gain1/1 -> Add6/3
  Gain4/1 -> Add6/4, Add7/1
  [DSup] -> Gain4/1
  Gain3/1 -> Add7/2
  Add5/1 -> Mux1/5
  Cast To Double/1 -> [DSup]

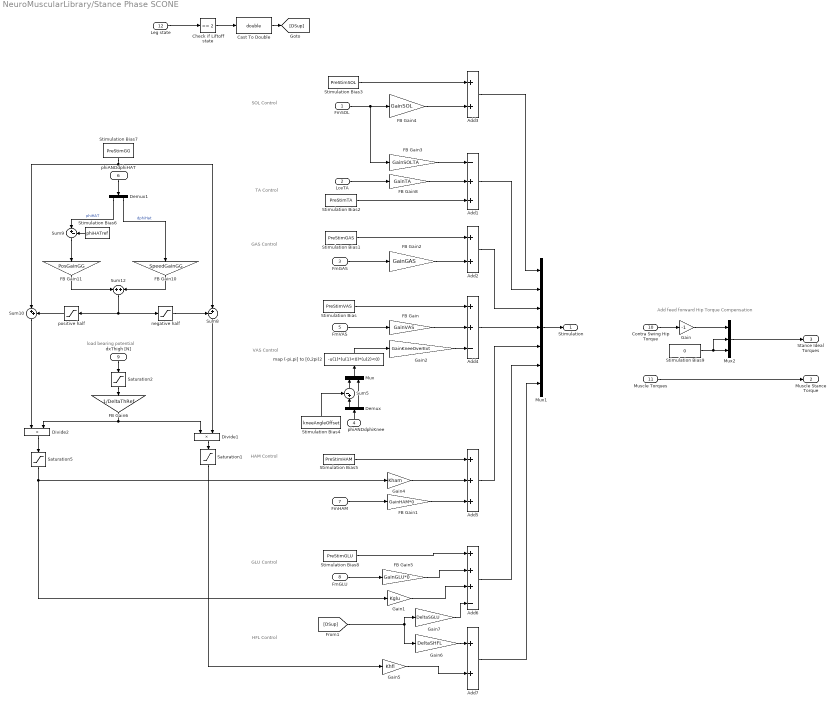
== system NeuroMuscularLibrary/Stance Phase SCONE ==
  note: Add feed forward Hip Torque Compensation
  note: load bearing potential
  note: HFL Control
  note: GLU Control
  note: VAS Control
  note: HAM Control
  note: GAS Control
  note: TA Control
  note: SOL Control
  FmSOL : Inport
  LceTA : Inport  Port=2
  FmGAS : Inport  Port=3
  phiANDdphiKnee : Inport  Port=4
  FmVAS : Inport  Port=5
  phiANDdphiHAT : Inport  Port=6
  FmHAM : Inport  Port=7
  FmGLU : Inport  Port=8
  dxThigh [N] : Inport  Port=9
  Contra Swing Hip Torque : Inport  Port=10
  Muscle Torques : Inport  Port=11
  Leg state : Inport  Port=12
  Add1 : Sum  Inputs=-++
  Add2 : Sum
  Add3 : Sum
  Add4 : Sum  Inputs=++-
  Add5 : Sum  Inputs=+++
  Add6 : Sum  Inputs=+++-
  Add7 : Sum
  Cast To Double : DataTypeConversion  OutDataTypeStr=double
  Check if Liftoff state : simulink/Logic and Bit Operations/Compare To Constant  relop===  const=2  OutDataTypeStr=boolean
  Demux : Demux  Outputs=2
  Demux1 : Demux  Outputs=2
  Divide1 : Product
  Divide2 : Product
  FB Gain : Gain  Gain=GainVAS  SaturateOnIntegerOverflow=on  OutDataTypeStr=Inherit: Same as input  ParamDataTypeStr=Inherit: Same as input
  FB Gain1 : Gain  Gain=GainHAM*0  SaturateOnIntegerOverflow=on  OutDataTypeStr=Inherit: Same as input  ParamDataTypeStr=Inherit: Same as input
  FB Gain10 : Gain  Gain=SpeedGainGG  SaturateOnIntegerOverflow=on  OutDataTypeStr=Inherit: Same as input  ParamDataTypeStr=Inherit: Same as input
  FB Gain11 : Gain  Gain=PosGainGG  SaturateOnIntegerOverflow=on  OutDataTypeStr=Inherit: Same as input  ParamDataTypeStr=Inherit: Same as input
  FB Gain2 : Gain  Gain=GainGAS  SaturateOnIntegerOverflow=on  OutDataTypeStr=Inherit: Same as input  ParamDataTypeStr=Inherit: Same as input
  FB Gain3 : Gain  Gain=GainSOLTA  SaturateOnIntegerOverflow=on  OutDataTypeStr=Inherit: Same as input  ParamDataTypeStr=Inherit: Same as input
  FB Gain4 : Gain  Gain=GainSOL  SaturateOnIntegerOverflow=on  OutDataTypeStr=Inherit: Same as input  ParamDataTypeStr=Inherit: Same as input
  FB Gain5 : Gain  Gain=GainGLU*0  SaturateOnIntegerOverflow=on  OutDataTypeStr=Inherit: Same as input  ParamDataTypeStr=Inherit: Same as input
  FB Gain6 : Gain  Gain=1/DeltaThRef  SaturateOnIntegerOverflow=on  OutDataTypeStr=Inherit: Same as input  ParamDataTypeStr=Inherit: Same as input
  FB Gain8 : Gain  Gain=GainTA  SaturateOnIntegerOverflow=on  OutDataTypeStr=Inherit: Same as input  ParamDataTypeStr=Inherit: Same as input
  Gain : Gain  Gain=-1
  Gain1 : Gain  Gain=Kglu
  Gain2 : Gain  Gain=GainKneeOverExt
  Gain4 : Gain  Gain=Kham
  Gain5 : Gain  Gain=Khfl
  Gain6 : Gain  Gain=DeltaSHFL
  Gain7 : Gain  Gain=DeltaSGLU
  Mux : Mux  Inputs=2
  Mux1 : Mux  Inputs=7
  Mux2 : Mux  Inputs=3
  Saturation1 : Saturate  UpperLimit=1  LowerLimit=0  ZeroCross=off
  Saturation2 : Saturate  UpperLimit=inf  LowerLimit=0  ZeroCross=off
  Saturation5 : Saturate  UpperLimit=1  LowerLimit=0  ZeroCross=off
  Stimulation Bias : Constant  Value=PreStimVAS
  Stimulation Bias1 : Constant  Value=PreStimGAS
  Stimulation Bias2 : Constant  Value=PreStimTA
  Stimulation Bias3 : Constant  Value=PreStimSOL
  Stimulation Bias4 : Constant  Value=kneeAngleOffset
  Stimulation Bias5 : Constant  Value=PreStimHAM
  Stimulation Bias6 : Constant  Value=phiHATref
  Stimulation Bias7 : Constant  Value=PreStimGG
  Stimulation Bias8 : Constant  Value=PreStimGLU
  Stimulation Bias9 : Constant  Value=0
  Sum10 : Sum  Inputs=|++  SaturateOnIntegerOverflow=on  InputSameDT=on  OutDataTypeStr=Inherit: Same as first input
  Sum12 : Sum  SaturateOnIntegerOverflow=on  InputSameDT=on  OutDataTypeStr=Inherit: Same as first input
  Sum5 : Sum  Inputs=-+|  SaturateOnIntegerOverflow=on  InputSameDT=on  OutDataTypeStr=Inherit: Same as first input
  Sum8 : Sum  Inputs=-+|  SaturateOnIntegerOverflow=on  InputSameDT=on  OutDataTypeStr=Inherit: Same as first input
  Sum9 : Sum  Inputs=|+-  SaturateOnIntegerOverflow=on  InputSameDT=on  OutDataTypeStr=Inherit: Same as first input
  map (-pi,pi] to [0,2pi)2 : Fcn  Expr=-u(1)*(u(1)<0)*(u(2)<0)
  negative half : Saturate  UpperLimit=0  LowerLimit=-inf  ZeroCross=off
  positive half : Saturate  UpperLimit=inf  LowerLimit=0  ZeroCross=off
  Stimulation : Outport
  Muscle Stance Torque : Outport  Port=2
  Stance Ideal Torques : Outport  Port=3
  wires:
  Gain/1 -> Mux2/1
  Contra Swing Hip Torque/1 -> Gain/1
  Add4/1 -> Mux1/4
  Mux1/1 -> Stimulation/1
  Gain1/1 -> Add6/3
  FB Gain5/1 -> Add6/2
  Stimulation Bias8/1 -> Add6/1
  Add6/1 -> Mux1/6
  Add5/1 -> Mux1/5
  FB Gain1/1 -> Add5/3
  Stimulation Bias5/1 -> Add5/1
  Stimulation Bias/1 -> Add4/1
  Stimulation Bias1/1 -> Add2/1
  Add2/1 -> Mux1/3
  Stimulation Bias2/1 -> Add1/3
  Stimulation Bias3/1 -> Add3/1
  FmGLU/1 -> FB Gain5/1
  FmHAM/1 -> FB Gain1/1
  map (-pi,pi] to [0,2pi)2/1 -> Gain2/1
  Sum8/1 -> Divide1/2
  Sum10/1 -> Divide2/1
  Sum9/1 -> FB Gain11/1
  FB Gain6/1 -> Divide1/1, Divide2/2
  Saturation5/1 -> Gain4/1, Gain1/1
  Divide2/1 -> Saturation5/1
  Divide1/1 -> Saturation1/1
  dxThigh [N]/1 -> Saturation2/1
  Saturation2/1 -> FB Gain6/1
  Saturation1/1 -> Gain5/1
  Gain2/1 -> Add4/3
  negative half/1 -> Sum8/1
  Sum12/1 -> negative half/1, positive half/1
  positive half/1 -> Sum10/2
  Demux1/2 -> FB Gain10/1  "dphiHat"
  Demux1/1 -> Sum9/1  "phiHAT"
  phiANDdphiHAT/1 -> Demux1/1
  FB Gain10/1 -> Sum12/2
  FB Gain11/1 -> Sum12/1
  Stimulation Bias7/1 -> Sum8/2, Sum10/1
  Stimulation Bias6/1 -> Sum9/2
  Stimulation Bias4/1 -> Sum5/1
  Demux/2 -> Mux/2
  Demux/1 -> Sum5/2
  phiANDdphiKnee/1 -> Demux/1
  Sum5/1 -> Mux/1
  Mux/1 -> map (-pi,pi] to [0,2pi)2/1
  FmVAS/1 -> FB Gain/1
  FB Gain/1 -> Add4/2
  FB Gain2/1 -> Add2/2
  FmGAS/1 -> FB Gain2/1
  LceTA/1 -> FB Gain8/1
  FB Gain8/1 -> Add1/2
  Add1/1 -> Mux1/2
  FB Gain3/1 -> Add1/1
  FmSOL/1 -> FB Gain3/1, FB Gain4/1
  FB Gain4/1 -> Add3/2
  Add3/1 -> Mux1/1
  Stimulation Bias9/1 -> Mux2/3, Mux2/2
  Mux2/1 -> Stance Ideal Torques/1
  Muscle Torques/1 -> Muscle Stance Torque/1
  Gain4/1 -> Add5/2
  Add7/1 -> Mux1/7
  Cast To Double/1 -> [DSup]
  Check if Liftoff state/1 -> Cast To Double/1
  Leg state/1 -> Check if Liftoff state/1
  [DSup] -> Gain7/1, Gain6/1
  Gain5/1 -> Add7/2
  Gain6/1 -> Add7/1
  Gain7/1 -> Add6/4

== system NeuroMuscularLibrary/Stance, Swing, Trans (coronal) ==
  note: DS1 (Stance -> Swing):
      | Stance Swing Transition
  note: Swing:
      | Swing Leg
  note: Full Stance:
      | PreStim, M3*F_i
  note: Stance DS1 Swing DS2
  note: FullStance Swing
  note: |------------------------------|--------------------|
  note: |--------------------|------------------------------|
  note: ContraSwing:
      | Swing Compensation
  Stance : Inport
  Contra Stance : Inport  Port=2
  Contra leg to leg : Inport  Port=3
  Ipsi lateral leg load : Inport  Port=4
  Contralateral leg load : Inport  Port=5
  S_0_St : Inport  Port=6
  S_M1 : Inport  Port=7
  S_M3 : Inport  Port=8
  S_M4 : Inport  Port=9
  S_0_Sw : Inport  Port=10
  S_M6 : Inport  Port=11
  Add : Sum  Inputs=4
  Add1 : Sum  Inputs=3
  Constant1 : Constant  Value=transsw_C
  Constant2 : Constant
  Constant5 : Constant  Value=transSupst_C
  Demux1 : Demux  Outputs=2
  Demux2 : Demux  Outputs=2
  Demux3 : Demux  Outputs=2
  Divide{1..2,4..5,12..15,24} (9 alike) : Product
  Divide31 : Product  Inputs=3
  Divide6 : Product  Inputs=3
  Logical Operator1 : Logic  Operator=NOT  AllPortsSameDT=off  OutDataTypeStr=boolean
  Logical Operator2 : Logic  Operator=NOT  AllPortsSameDT=off  OutDataTypeStr=boolean
  Logical Operator5 : Logic  Operator=NOT  AllPortsSameDT=off  OutDataTypeStr=boolean
  Logical Operator7 : Logic  AllPortsSameDT=off  OutDataTypeStr=boolean
  Mux3 : Mux  Inputs=2
  Sum1 : Sum  Inputs=|++  SaturateOnIntegerOverflow=on  InputSameDT=on  OutDataTypeStr=Inherit: Same as first input
  Sum2 : Sum  Inputs=|++  SaturateOnIntegerOverflow=on  InputSameDT=on  OutDataTypeStr=Inherit: Same as first input
  Sum4 : Sum  SaturateOnIntegerOverflow=on  InputSameDT=on  OutDataTypeStr=Inherit: Same as first input
  Sum5 : Sum  Inputs=+-|  SaturateOnIntegerOverflow=on  InputSameDT=on  OutDataTypeStr=Inherit: Same as first input
  Sum6 : Sum  Inputs=++|  SaturateOnIntegerOverflow=on  InputSameDT=on  OutDataTypeStr=Inherit: Same as first input
  S : Outport  OutputWhenDisabled=reset  InitialOutput=0
  wires:
  Contra Stance/1 -> Logical Operator1/1
  S_M4/1 -> Divide15/2
  Logical Operator1/1 -> Divide15/1
  Contralateral leg load/1 -> Divide1/2, Divide24/1
  Divide1/1 -> Divide31/2
  Contra leg to leg/1 -> Logical Operator5/1, Divide31/1, Divide14/1  "double support"
  Stance/1 -> Logical Operator2/1, Divide6/1, Divide4/1, Logical Operator7/1
  Logical Operator2/1 -> Divide2/1, Divide5/1
  Add/1 -> Mux3/1
  Add1/1 -> Mux3/2
  S_M3/1 -> Divide6/2
  Ipsi lateral leg load/1 -> Divide6/3
  S_0_St/1 -> Divide4/2
  S_0_Sw/1 -> Divide5/2
  Mux3/1 -> Sum6/2
  Sum6/1 -> S/1
  S_M6/1 -> Divide31/3, Divide2/2
  Divide4/1 -> Sum4/1, [M0_St]  "M0_St (1~2)"
  Divide5/1 -> Sum4/2, [M0_Sw]  "M0_Sw (3~4)"
  Divide31/1 -> Sum1/1
  Divide2/1 -> Sum1/2
  S_M1/1 -> Divide12/2, Divide13/1  "HAB"
  Divide12/1 -> Sum2/1
  Divide13/1 -> Divide14/2
  Divide14/1 -> Sum2/2
  Logical Operator5/1 -> Logical Operator7/2
  Logical Operator7/1 -> Divide12/1  "single stance"
  Divide24/1 -> Sum5/2
  Constant2/1 -> Sum5/1
  Sum5/1 -> Divide13/2
  Constant5/1 -> Divide24/2  "Tr_St_sup"
  Constant1/1 -> Divide1/1  "Tr_Sw"
  Sum2/1 -> [M1_HAB]
  Divide6/1 -> Demux3/1
  Demux3/1 -> [M3_HAB]
  Demux3/2 -> [M3_HAD]
  Divide15/1 -> Demux1/1
  Demux1/1 -> [M4_HAB]
  Demux1/2 -> [M4_HAD]
  Demux2/1 -> [M6_HAB]
  Demux2/2 -> [M6_HAD]
  Sum1/1 -> Demux2/1
  Sum4/1 -> Sum6/1
  [M1_HAB] -> Add/1
  [M3_HAB] -> Add/2
  [M3_HAD] -> Add1/1
  [M4_HAB] -> Add/3
  [M6_HAB] -> Add/4
  [M4_HAD] -> Add1/2
  [M6_HAD] -> Add1/3
